simulink model "bluetoothcel2"  (R2020a)
settings: Solver=FixedStepAuto  StartTime=0.0  StopTime=10.0  RelTol=1e-3
undefined symbols (not defined in the file): F2, F5, F8
libraries: androiduilib x5, simulink x4, androidaudiovideolib x2, androidcommunicationlib x2, dspswit3 x1, androidsensorlib x1
settings Model: Creator=luisi  LastModifiedBy=luisi
settings OptimizationCC: EnhancedBackFolding=on  PassReuseOutputArgsAs=Individual arguments  ZeroExternalMemoryAtStartup=off  ZeroInternalMemoryAtStartup=off  MaxStackSize=64  OptimizeBlockOrder=speed  DifferentSizesBufferReuse=on  OptimizationCustomize=off  EfficientTunableParamExpr=on
settings DebuggingCC: ParameterTunabilityLossMsg=error
settings HardwareCC: ProdBitPerPointer=32  ProdBitPerSizeT=32  ProdBitPerPtrDiffT=32  ProdLargestAtomicInteger=Long  ProdLargestAtomicFloat=Double  ProdWordSize=32  ProdHWDeviceType=ARM Compatible->ARM Cortex
settings SFSimCC: MATLABDynamicMemAlloc=off
settings RTWCC: SystemTargetFile=ert.tlc  HardwareBoard=Android Device  TemplateMakefile=ert_default_tmf  RTWVerbose=off  Toolchain=Android SDK/NDK Tools
settings CodeAppCC: ForceParamTrailComments=on  IgnoreCustomStorageClasses=off  OperatorAnnotations=on  SimulinkDataObjDesc=on  SFDataObjDesc=on  InsertBlockDesc=on
settings ERTTargetCC: ExtModeMexArgs='localhost'

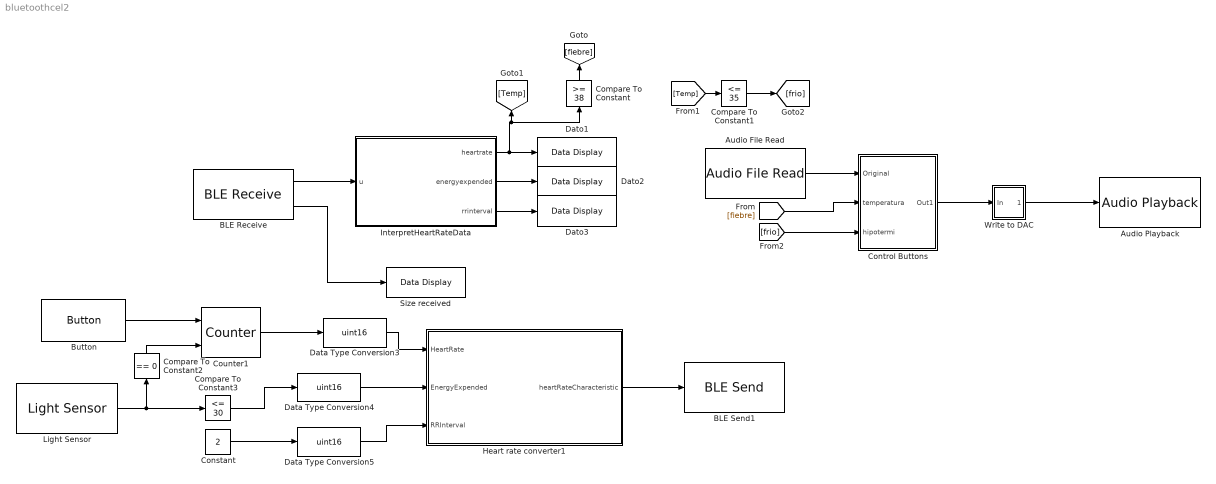
== system bluetoothcel2 ==
  Audio File Read : androidaudiovideolib/Audio File Read  FileName=C:\Users\luisi\Downloads\baby.mp3  FrameSize=4410
      settings: SourceProductBaseCode=ANDROID
  Audio Playback : androidaudiovideolib/Audio Playback  SampleFreq=44100  AudioSamplingFreq=44100  SampleTime=0.1  DeviceStr=0  QueueDuration=0  BlockPlatform=Android
      settings: SourceProductBaseCode=ANDROID
  BLE Receive : androidcommunicationlib/BLE Receive  DeviceMode=Central (Client)  BluetoothAddress=54:F2:63:F5:F8:7B  CharUUID=00002a37-0000-1000-8000-00805f9b34fb  ServiceUUID=0000180d-0000-1000-8000-00805f9b34fb  device=RedmiLuisa  character="Heart Rate\\Heart Rate  Measurement"  CustomService=off  ServiceName=Heart Rate  CharacteristicName="Heart Rate  Measurement"  CustomServiceUUID=<Enter Service UUID>  CustomCharUUID=<Enter Characteristic UUID>  DataSize=7  SampleTime=0.1  charseruuid=00001801-0000-1000-8000-00805f9b34fb\00002a05-0000-1000-8000-00805f9b34fb  seruuid=00001810-0000-1000-8000-00805f9b34fb  PeripheralService=0000180d-0000-1000-8000-00805f9b34fb  PeripheralCharacteristic=00002a37-0000-1000-8000-00805f9b34fb  chruuid=00002a37-0000-1000-8000-00805f9b34fb  BLEId=bluetoothcel2/BLE_Receive  Devicename=RedmiLuisa  IsCustomService=0
      settings: SourceProductBaseCode=ANDROID
  BLE Send1 : androidcommunicationlib/BLE Send  DeviceMode=Peripheral (Server)  BluetoothAddress=54:F2:63:F5:F8:7B  CharUUID=00002a05-0000-1000-8000-00805f9b34fb  ServiceUUID=00001801-0000-1000-8000-00805f9b34fb  device=RedmiLuisa  character=Generic Attribute\Service Changed  CustomService=off  ServiceName=Heart Rate  CharacteristicName="Heart Rate  Measurement"  CustomServiceUUID=<Enter Service UUID>  CustomCharUUID=<Enter Characteristic UUID>  charseruuid=00001801-0000-1000-8000-00805f9b34fb\00002a05-0000-1000-8000-00805f9b34fb  seruuid=00001810-0000-1000-8000-00805f9b34fb  chruuid=00002a37-0000-1000-8000-00805f9b34fb  PeripheralService=0000180d-0000-1000-8000-00805f9b34fb  PeripheralCharacteristic=00002a37-0000-1000-8000-00805f9b34fb  BLEId=bluetoothcel2/BLE_Send1  Devicename=RedmiLuisa  IsCustomService=0  Size=-1
      settings: SourceProductBaseCode=ANDROID
  Button : androiduilib/Button  ButtonState=Not pressed  ButtonId=bluetoothcel2/Button  State=off  SampleTime=0.1  BlockPlatform=Android
      settings: SourceProductBaseCode=ANDROID
  Compare To Constant : simulink/Logic and Bit Operations/Compare To Constant  relop=>=  const=38  OutDataTypeStr=boolean
  Compare To Constant1 : simulink/Logic and Bit Operations/Compare To Constant  relop=<=  const=35  OutDataTypeStr=boolean
  Compare To Constant2 : simulink/Logic and Bit Operations/Compare To Constant  relop===  const=0  OutDataTypeStr=boolean
  Compare To Constant3 : simulink/Logic and Bit Operations/Compare To Constant  relop=<=  const=30  OutDataTypeStr=boolean
  Constant : Constant  Value=2
  Control Buttons : Subsystem
  Counter1 : dspswit3/Counter  Direction=Up  CountEvent=Rising edge  CounterSize=User defined  MaxCount=100  InitialCount=0  Output=Count  HitValue=32  ResetInput=on  SamplesPerFrame=1  Ts=1  CntDtype=double  HitDtype=Logical
  Data Type Conversion3 : DataTypeConversion  OutDataTypeStr=uint16
  Data Type Conversion4 : DataTypeConversion  OutDataTypeStr=uint16
  Data Type Conversion5 : DataTypeConversion  OutDataTypeStr=uint16
  Dato1 : androiduilib/Data Display  DataDisplayId=bluetoothcel2/Dato1  Format=Float  Precision=6  SimulateUsing=Code generation  blockPlatform=Android
      settings: SourceProductBaseCode=ANDROID
  Dato2 : androiduilib/Data Display  DataDisplayId=bluetoothcel2/Dato2  Format=Float  Precision=6  SimulateUsing=Code generation  blockPlatform=Android
      settings: SourceProductBaseCode=ANDROID
  Dato3 : androiduilib/Data Display  DataDisplayId=bluetoothcel2/Dato3  Format=Float  Precision=6  SimulateUsing=Code generation  blockPlatform=Android
      settings: SourceProductBaseCode=ANDROID
  Heart rate converter1 : MATLAB Function  TreatAsAtomicUnit=on
  InterpretHeartRateData : MATLAB Function  TreatAsAtomicUnit=on
  Light Sensor : androidsensorlib/Light Sensor  SampleTime=0.1  BlockPlatform=Android
      settings: SourceProductBaseCode=ANDROID
  Size received : androiduilib/Data Display  DataDisplayId=bluetoothcel2/Size_received  Format=Float  Precision=6  SimulateUsing=Code generation  blockPlatform=Android
      settings: SourceProductBaseCode=ANDROID
  Write to DAC : Subsystem
  wires:
  Constant/1 -> Data Type Conversion5/1
  Data Type Conversion4/1 -> Heart rate converter1/2(EnergyExpended)
  Compare To Constant3/1 -> Data Type Conversion4/1
  Heart rate converter1/1(heartRateCharacteristic) -> BLE Send1/1
  Counter1/1 -> Data Type Conversion3/1
  BLE Receive/2 -> Size received/1
  Data Type Conversion3/1 -> Heart rate converter1/1(HeartRate)
  Data Type Conversion5/1 -> Heart rate converter1/3(RRInterval)
  InterpretHeartRateData/3(rrinterval) -> Dato3/1
  BLE Receive/1 -> InterpretHeartRateData/1(u)
  InterpretHeartRateData/2(energyexpended) -> Dato2/1
  Audio File Read/1 -> Control Buttons/1(Original)
  [fiebre] -> Control Buttons/2(temperatura)
  Control Buttons/1(Out1) -> Write to DAC/1(In)
  [frio] -> Control Buttons/3(hipotermi)
  Light Sensor/1 -> Compare To Constant3/1, Compare To Constant2/1
  [Temp] -> Compare To Constant1/1
  Button/1 -> Counter1/1
  Compare To Constant2/1 -> Counter1/2
  Compare To Constant/1 -> [fiebre]
  Write to DAC/1(Out) -> Audio Playback/1
  InterpretHeartRateData/1(heartrate) -> Dato1/1, Compare To Constant/1, [Temp]
  Compare To Constant1/1 -> [frio]

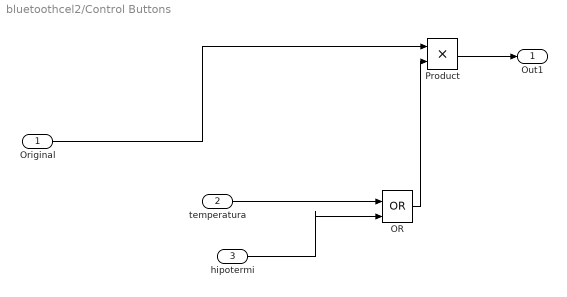
== system bluetoothcel2/Control Buttons ==
  Original : Inport
  temperatura : Inport  Port=2
  hipotermi : Inport  Port=3
  OR : Logic  Operator=OR  IconShape=distinctive  AllPortsSameDT=off  OutDataTypeStr=boolean
  Product : Product
  Out1 : Outport  VectorParamsAs1DForOutWhenUnconnected=off
  wires:
  Product/1 -> Out1/1
  Original/1 -> Product/1
  temperatura/1 -> OR/1
  hipotermi/1 -> OR/2
  OR/1 -> Product/2

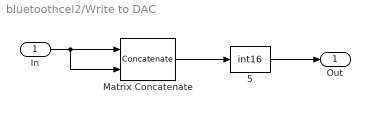
== system bluetoothcel2/Write to DAC ==
  In : Inport
  " 5" : DataTypeConversion  OutDataTypeStr=int16
  Matrix Concatenate : Concatenate  Mode=Multidimensional array  ConcatenateDimension=2
  Out : Outport  VectorParamsAs1DForOutWhenUnconnected=off
  wires:
  In/1 -> Matrix Concatenate/2, Matrix Concatenate/1
  Matrix Concatenate/1 -> " 5"/1
  " 5"/1 -> Out/1

== matlab function bluetoothcel2/InterpretHeartRateData ==
  data: u input; heartrate output; energyexpended output; rrinterval output
function [heartrate, energyexpended, rrinterval ] = InterpretHeartRateData(u)
flag = uint8(u(1));
heartrate = uint16(0);
energyexpended=uint16(0);
rrinterval = uint16(0);
b = bitget(flag,8:-1:1);

 if b(8) == 0
     format = uint8(2);
     heartrate = uint16(u(2));
 else
     format = uint8(3);
     heartrate = typecast([u(2) u(3)], 'uint16');
 end
 
 if b(5) == 1
     energy = uint8(2);
     energyexpended = typecast([u(format +1) u(format + 2)], 'uint16');
 else
     energy = uint8(0);
     energyexpended = uint16(0);
 end
 
 if b(4) == 1
     rrinterval = typecast([u(format +energy + 1) u(format + energy + 2)],'uint16');
 else
     rrinterval = uint16(0);
 end
end

== matlab function bluetoothcel2/Heart rate converter1 ==
  data: HeartRate input; heartRateCharacteristic output; EnergyExpended input; RRInterval input
function heartRateCharacteristic = ConvertToHeartRateFormat(HeartRate, EnergyExpended, RRInterval)
flag = uint8(25);
heartRateCharacteristic = zeros(7,1,'uint8');
heartRateCharacteristic(1)= flag;
[lower, upper] = getBytes(HeartRate);
heartRateCharacteristic(2) = lower;
heartRateCharacteristic(3) = upper;
[lower, upper] = getBytes(EnergyExpended);
heartRateCharacteristic(4) = lower;
heartRateCharacteristic(5) = upper;
[lower, upper] = getBytes(RRInterval);
heartRateCharacteristic(6) = lower;
heartRateCharacteristic(7) = upper;
end

function [lower,upper] = getBytes(parameter)
h = dec2bin(parameter,16);
lower = bin2dec(h(9:16));
upper= bin2dec(h(1:8));
end
